simulink model "c2000_host_CAN_comm"  (R2021b)
settings: Solver=VariableStepAuto  StartTime=0.0  StopTime=Inf  RelTol=1e-3  EnableMultiTasking=on
undefined symbols (not defined in the file or in its folder): canChannel
libraries: canlib x3, canmsglib x2, demo_controls x1, simulink x1
settings Model: ExtModeTrigDuration=8  Creator=The MathWorks, Inc.  LastModifiedBy=The MathWorks, Inc.
settings SolverCC: AlgebraicLoopSolver=TrustRegion
settings DebuggingCC: SFMachineParentedDataDiag=warning

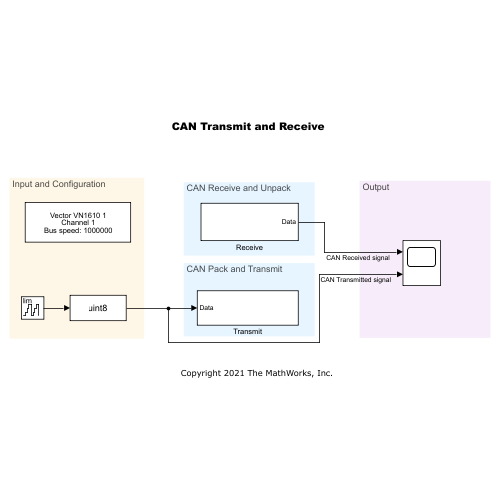
[thumbnail: Simulink's stored preview of the top-level diagram]
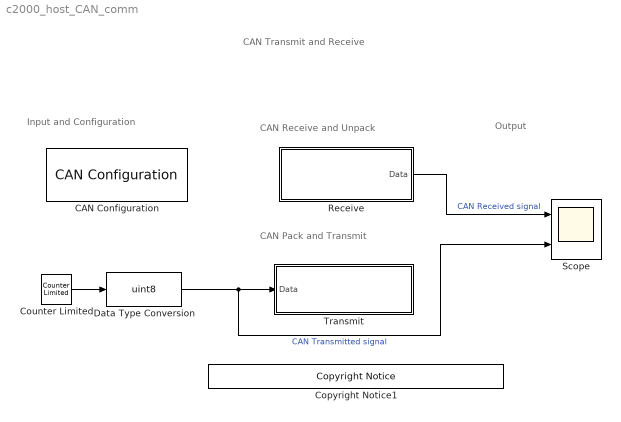
== system c2000_host_CAN_comm ==
  note: CAN Transmit and Receive
  note: Input and Configuration
  note: Output
  note: CAN Receive and Unpack
  note: CAN Pack and Transmit
  CAN Configuration : canlib/CAN Configuration  BlockHandle=2.015  Device=MathWorks Virtual 1 (Channel 1)  DeviceMenu=MathWorks Virtual 1 (Channel 1)  ObjConstructor=canChannel('MathWorks', 'Virtual 1', 1)  BusSpeed=1000000  EnableBitParameters=off  SJW=1  TSEG1=4  TSEG2=3  NSamples=1  AckMode=Normal
      settings: SourceProductBaseCode=VN
  Copyright Notice1 : demo_controls/Copyright Notice  year=2021  prod=tic2000
      settings: SourceProductBaseCode=ME
  Counter Limited : simulink/Sources/Counter Limited  uplimit=255  tsamp=0.05
  Data Type Conversion : DataTypeConversion  OutDataTypeStr=uint8
  Receive : Subsystem  Priority=40
  Scope : Scope  NumInputPorts=2
  Transmit : Subsystem  Priority=30
  wires:
  Data Type Conversion/1 -> Scope/2, Transmit/1(Data)  "CAN Transmitted signal"
  Counter Limited/1 -> Data Type Conversion/1
  Receive/1(Data) -> Scope/1  "CAN Received signal"

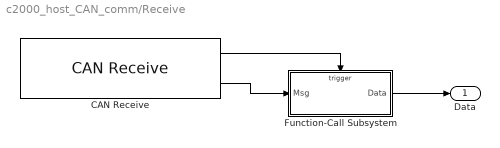
== system c2000_host_CAN_comm/Receive ==
  CAN Receive : canlib/CAN Receive  BlockHandle=7.015  Device=MathWorks Virtual 1 (Channel 1)  DeviceMenu=MathWorks Virtual 1 (Channel 1)  ObjConstructor=canChannel('MathWorks', 'Virtual 1', 1)  EnableStandardIDsFilter=off  StdIDsCombo=Allow only  StandardIDs=hex2dec('0x0000000C')  EnableExtendedIDsFilter=off  ExtIDsCombo=Block all  ExtendedIDs=hex2dec('0x0000C000')  SampleTime=0.05  MsgsPerTimestep=all  InternalFilterUpdateStatus=on  BusOutput=off
      settings: SourceProductBaseCode=VN
  Function-Call Subsystem : Subsystem  TreatAsAtomicUnit=on
  Data : Outport
  wires:
  CAN Receive/1 -> Function-Call Subsystem/Trigger
  CAN Receive/2 -> Function-Call Subsystem/1(Msg)
  Function-Call Subsystem/1(Data) -> Data/1

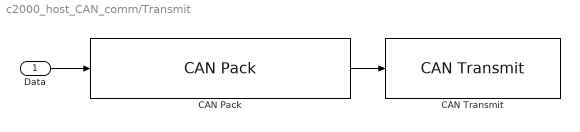
== system c2000_host_CAN_comm/Transmit ==
  Data : Inport
  CAN Pack : canmsglib/CAN Pack  MsgList=(none)  MsgName=CAN Msg  MsgIDType=Standard (11-bit identifier)  MsgIdentifier=hex2dec('0x0000037B')  MsgLength=1  Remote=off  ApplyMinMax=off  BusOutput=off  SignalInfo={}
      settings: SourceProductBaseCode=ME,XP,VN  DataFormat=raw data
  CAN Transmit : canlib/CAN Transmit  BlockHandle=23.0166  Device=MathWorks Virtual 1 (Channel 1)  DeviceMenu=MathWorks Virtual 1 (Channel 1)  ObjConstructor=canChannel('MathWorks', 'Virtual 1', 1)  EnableEventTransmit=on  EnablePeriodicTransmit=off  MessagePeriod=0.005
      settings: SourceProductBaseCode=VN
  wires:
  CAN Pack/1 -> CAN Transmit/1
  Data/1 -> CAN Pack/1

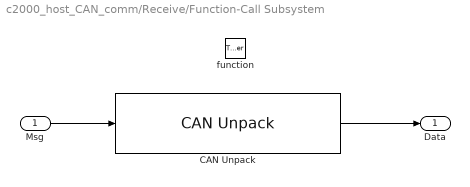
== system c2000_host_CAN_comm/Receive/Function-Call Subsystem ==
  Msg : Inport
  function : TriggerPort  TriggerType=function-call  VariantControl=(inherit)
  CAN Unpack : canmsglib/CAN Unpack  MsgList=(none)  MsgName=CAN Msg  MsgIDType=Standard (11-bit identifier)  MsgIdentifier=hex2dec('0x0000000C')  MsgLength=1  SignalInfo={}  IDPort=off  TimestampPort=off  ErrorPort=off  RemotePort=off  LengthPort=off  StatusPort=off  ApplyMinMax=off
      settings: SourceProductBaseCode=ME,XP,VN  DataFormat=raw data
  Data : Outport
  wires:
  CAN Unpack/1 -> Data/1
  Msg/1 -> CAN Unpack/1
